simulink model "VTOL_v2"  (R2019b)
settings: Solver=FixedStepAuto  StartTime=0.0  StopTime=inf  FixedStep=Ts  RelTol=1e-3  EnableMultiTasking=on
values from neighbouring files (symbols this model uses):
  k1 = (0.5/axisgains(2) - k2*cruiseThrottle^2)/(cruiseVel^2)    [SensitivityParameterFinder.m]
  k2 = 0.5/(axisgains(2)*hoverpower(1).^2)    [SensitivityParameterFinder.m]
  k3 = (0.5/axisgains(1) - k4*cruiseThrottle^2)/(cruiseVel^2)    [SensitivityParameterFinder.m]
  k4 = 0.5/(axisgains(1)*hoverpower(1).^2)    [SensitivityParameterFinder.m]
  Ts = 1/100    (= 0.01)    [VTOL_params.m]
undefined symbols (not defined in the file or in its folder): color, deltaprops, dev, led_mask, Main, mode, MRC, pwm_output0
libraries: px4uORBlib x13, aerolibutil x8, simulink x6, pwm_sig_converters x4, px4Sensorslib x2, px4lib x2, sharedtransform x2
(part 1 of 3)
settings Model: SimulationMode=external  ExtModeTrigDuration=10  Creator=Robert  LastModifiedBy=Robert
settings SolverCC: PositivePriorityOrder=on  AutoInsertRateTranBlk=on
settings DataIOCC: SaveOutput=off  SignalLogging=off  DSMLogging=off  SaveTime=off  ReturnWorkspaceOutputs=off
settings OptimizationCC: DefaultUnderspecifiedDataType=single  EnhancedBackFolding=on  PassReuseOutputArgsAs=Individual arguments  MaxStackSize=64  OptimizeBlockOrder=speed  DifferentSizesBufferReuse=on  OptimizationCustomize=off  EfficientTunableParamExpr=on
settings DebuggingCC: ParameterTunabilityLossMsg=error  ArithmeticOperatorsInVariantConditions=warning
settings HardwareCC: ProdBitPerPointer=32  ProdBitPerSizeT=32  ProdBitPerPtrDiffT=32  ProdLargestAtomicInteger=Long  ProdLargestAtomicFloat=Double  ProdWordSize=32  ProdLongLongMode=on  ProdHWDeviceType=ARM Compatible->ARM Cortex
settings SFSimCC: MATLABDynamicMemAlloc=off  CustomCodeUndefinedFunction=UseInterfaceOnly
settings RTWCC: SystemTargetFile=ert.tlc  HardwareBoard=PX4 Pixhawk 1  TLCOptions="-aInlineSetEventsForThisBaseRateFcn=TLC_FALSE -aSuppressMultiTaskScheduler=TLC_FALSE  -aRateBasedStepFcn=0"  TemplateMakefile=ert_default_tmf  GenerateReport=on  Toolchain=GNU Tools for PX4 Autopilots  BuildConfiguration=Faster Runs  IncludeHyperlinkInReport=on  LaunchReport=on  TargetLang=C++  GenerateTraceInfo=on  GenerateTraceReport=on  GenerateTraceReportSl=on  GenerateTraceReportSf=on  GenerateTraceReportEml=on
settings CodeAppCC: ForceParamTrailComments=on  IgnoreCustomStorageClasses=off  OperatorAnnotations=on  SimulinkDataObjDesc=on  SFDataObjDesc=on  InsertBlockDesc=on
settings ERTTargetCC: ExtMode=on  ExtModeMexArgs='127.0.0.1' 1 17725

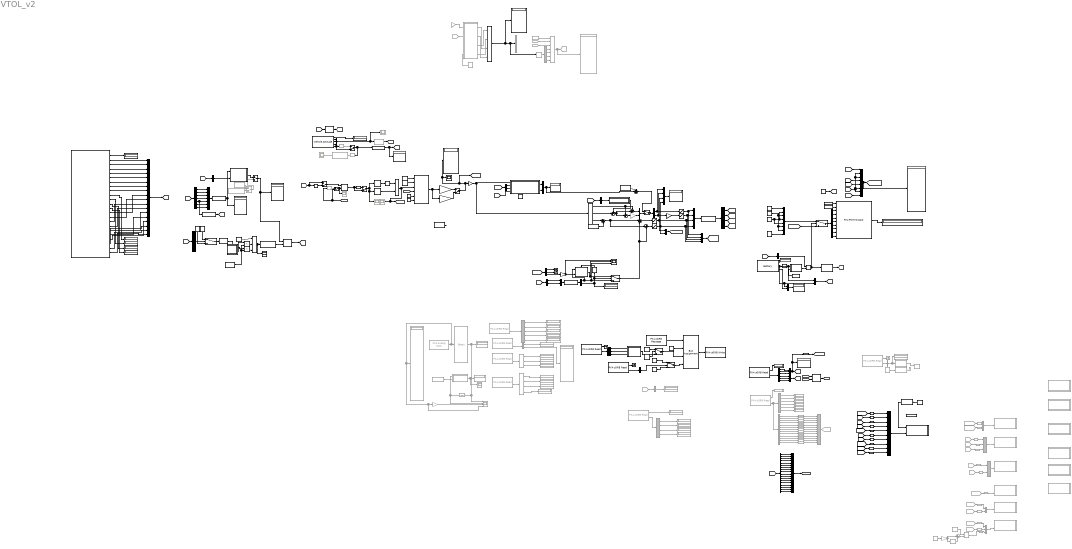
== system VTOL_v2 ==
  note: If SC is touched, initiate step sequence in roll and pitch.
  note: The above needs to match selection in next area;
      | if you run without torque-translator use the top,
      | else the bottom.
  note: Hover requires roughly 0.28 in TL/TR signals.
  note: Old log blocks, MW have given the custgom new ones
  note: The PID parameters for roll/pitch on the single engine one
      | that works are approx
      | [0.6,0,0.015;
      |  0.6,0,0.015]
      |
      | That is, P/D = 40
  note: Some constant pitch torque offset
      | may be necessary due to c.g. z-offset. (No integrators in controller)
  note: Control Area
  note: Before Torque-Translator is used, lets make sure we can hover with this simple linear mixer.
      | Working around the hover point does not need the full range and thus complete non-linear controller.
      | Basic tuning is easier this way - less parameters to adjust.
  note: Part 2 of 2 of the heart of this project.
      | Once the Pixhawk is stable and hover works acceptable this part will be inserted, normalized to not
      | alter the behaviour too much at hover mode, and extend the responses to work well in flying and
      | transition mode as well.
  note: Old translator, only kept for code reference, will never be used.
  note: Crude, ad-hoc, altitude holder for the hover mode.
      | Far from perfect but does the job and frees up one hand to trim/adjust setting etc while hovering.
      | When not holding alt => Pass through
      | throttle stick to joint thrust.
  note: Generate reference quaternion from Transmitter inputs. Very crude reference now, but enough to test stability and do some small steps.
      | Verified in external mode with manual switches.
      |
      | The "mode" (bottom) selects absolute/rate mode
      | on input..
  note: Quaternion extraction from EKF.
      | Handedness verified with manual switches in external mode.
  note: Debug safety switch status
  note: lowpass filter batt voltage for
      | more accurate shutoffs
  note: 3V/cell in LiPo is absolutely the lowest allowed
  note: Make sure model runs at specified frequency
  note: Above (commented out) was a work-around before I got the
      | fixed code for the log block to log at every time step.
  note: Props may not be symmetrical, this offsets the thrust to compensate in that case.
  note: Emergency shutdown switch forces things into
      | off or neutral
  note: Inputs from RC
  note: Outputs, to Servos
  note: Emil Fresk paper on quaternion control, this is part 1 of 2 of the focus on this project. Originally a non-linear attitude controller for
      | multi-rotors, I am trying to use it as a controller for a VTOL fixed wing, non vectored along with a sensitivity normalizer
      | to allow a single controller for hover, transitioning and flying modes.
  note: If either manual emergency stop is pressed or voltage too low cut power.
  note: Logging to SD
  note: Blink LED slowly with Green color on Pixhawk 1
  AND : Logic  Commented=on  IconShape=distinctive  AllPortsSameDT=off  OutDataTypeStr=boolean
  Battery : px4Sensorslib/Battery  voltage=on  current=off  remaining=on  warning=off  timestamp=off  sampleTime=Ts  BlockingMode=off  BlockTimeout=1e-3
      settings: SourceProductName=Embedded Coder Support Package for PX4 Autopilots
  Blink Fast : Constant  Value=5  OutDataTypeStr=Inherit: Inherit via back propagation  SampleTime=1
  Blink Slow : Constant  Value=3  OutDataTypeStr=Inherit: Inherit via back propagation  SampleTime=1
  Bus Assignment : BusAssignment  AssignedSignals=led_mask,color,mode
  Bus Creator : BusCreator  Inputs=18
  Bus Selector : BusSelector  Commented=on  OutputSignals=ch9_SC
  Bus Selector1 : BusSelector  Commented=on  OutputSignals=safety_switch_available,safety_off,override_available,override_enabled
  Bus Selector10 : BusSelector  Commented=on  OutputSignals=fix_type,satellites_used,lat,lon,alt,hdop,vdop,noise_per_ms,jamming_indicator,vel_m_s,vel_n_m_s,vel_e_m_s,vel_d_m_s
  Bus Selector11 : BusSelector  OutputSignals=ch10_SD
  Bus Selector12 : BusSelector  OutputSignals=ch5_S1
  Bus Selector13 : BusSelector  Commented=on  OutputSignals=safety_off
  Bus Selector14 : BusSelector  Commented=on  OutputSignals=channel_value,channel_id
  Bus Selector15 : BusSelector  Commented=on  OutputSignals=hdop,vdop,satellites_used
  Bus Selector16 : BusSelector  Commented=on  OutputSignals=differential_pressure_raw_pa,differential_pressure_filtered_pa,temperature,device_id
  Bus Selector17 : BusSelector  OutputSignals=ch9_SC
  Bus Selector18 : BusSelector  OutputSignals=satellites_used,hdop,vdop
  Bus Selector2 : BusSelector  OutputSignals=ch5_S1
  Bus Selector3 : BusSelector  OutputSignals=ch1_thrust,ch2_Ail,ch3_Ele,ch4_Rud,ch8_SB,ch6_S2,ch7_SA
  Bus Selector4 : BusSelector  OutputSignals=safety_off
  Bus Selector5 : BusSelector  Commented=on  OutputSignals=indicated_airspeed_m_s,true_airspeed_m_s,true_airspeed_unfiltered_m_s,confidence,air_temperature_celsius
  Bus Selector6 : BusSelector  OutputSignals=x,y,z,vx,vy,vz
  Bus Selector7 : BusSelector  OutputSignals=ch1_thrust,ch2_Ail,ch3_Ele,ch4_Rud,ch5_S1,ch6_S2,ch7_SA,ch8_SB,ch9_SC,ch10_SD,ch11_SE,ch12_SF,ch13_SG,ch14_SH,ch15_LS,ch16_RS,ch17_MAX,ch18_MIN
  Bus Selector8 : BusSelector  Commented=on  OutputSignals=lat,lon,alt,satellites_used,hdop,vdop
  Bus Selector9 : BusSelector  OutputSignals=ch1_thrust,ch12_SF
  Cast To Boolean : DataTypeConversion  Commented=on  OutDataTypeStr=boolean
  Cast To Boolean1 : DataTypeConversion  OutDataTypeStr=boolean
  Cast To Boolean2 : DataTypeConversion  OutDataTypeStr=boolean
  Color Amber : Constant  Value=6  OutDataTypeStr=Inherit: Inherit via back propagation  SampleTime=1
  Color Green : Constant  Value=2  OutDataTypeStr=Inherit: Inherit via back propagation  SampleTime=1
  Compare To Zero : simulink/Logic and Bit Operations/Compare To Zero  relop=>  OutDataTypeStr=boolean
  Constant : Constant  Value=logical(1)
  Constant1 : Constant  Value=logical(0)
  Constant10 : Constant  Value=1500  OutDataTypeStr=uint16
  Constant11 : Constant  Value=1500  OutDataTypeStr=uint16
  Constant12 : Constant  Value=1500  OutDataTypeStr=uint16  SampleTime=Ts
  Constant13 : Constant  Commented=on  Value=[cos(pi/4),0,sin(pi/4),0]  SampleTime=Ts
  Constant14 : Constant  Value=boolean(true)  SampleTime=Ts
  Constant15 : Constant  Value=255  OutDataTypeStr=Inherit: Inherit via back propagation  SampleTime=1
  Constant16 : Constant  Commented=on  SampleTime=Ts
  Constant17 : Constant  Value=[3.4,3.4,0.7]'  VectorParams1D=off  SampleTime=Ts
  Constant18 : Constant  Value=0.3  SampleTime=Ts
  Constant19 : Constant  Value=0.6  SampleTime=Ts
  Constant2 : Constant  Commented=on  Value=[0,0,0]  OutDataTypeStr=single  SampleTime=Ts
  Constant20 : Constant  Value=0*0.17.*[1,-1]
  Constant21 : Constant  Commented=on  Value=1.324
  Constant22 : Constant  Value=deg2rad(30)  OutDataTypeStr=single  SampleTime=Ts
  Constant23 : Constant  OutDataTypeStr=single  SampleTime=Ts
  Constant24 : Constant  Value=0  OutDataTypeStr=single  SampleTime=Ts
  Constant25 : Constant  Value=0  OutDataTypeStr=single  SampleTime=Ts
  Constant3 : Constant  Commented=on  Value=0  SampleTime=Ts
  Constant4 : Constant  Value=0.1  SampleTime=Ts
  Constant5 : Constant  Value=0.6  SampleTime=Ts
  Constant6 : Constant  Value=[0,0,0]  SampleTime=Ts
  Constant7 : Constant  Value=1500  OutDataTypeStr=uint16
  Constant8 : Constant  Commented=on  Value=[1,0,0,0]  SampleTime=Ts
  Constant9 : Constant  Value=900  OutDataTypeStr=uint16
  Counter Free-Running : simulink/Sources/Counter Free-Running  Commented=on  NumBits=16  tsamp=Ts
  CutoffVoltage : Constant  Value=3.0*3  OutDataTypeStr=single  SampleTime=Ts
  Data Type Conversion{1..16,20..26,28} (24 alike) : DataTypeConversion  Commented=on  OutDataTypeStr=single
  Data Type Conversion{17,29..30,32..34,36..39,41} (11 alike) : DataTypeConversion  OutDataTypeStr=single
  Data Type Conversion18 : DataTypeConversion  Commented=on  OutDataTypeStr=uint16
  Data Type Conversion19 : DataTypeConversion  Commented=on  OutDataTypeStr=uint16
  Data Type Conversion27 : DataTypeConversion  Commented=on  OutDataTypeStr=double
  Demux : Demux  Outputs=8
  Demux1 : Demux  Commented=on
  Demux2 : Demux  Outputs=2
  Demux4 : Demux  Commented=on
  Demux5 : Demux  Outputs=3
  Demux6 : Demux  Outputs=2
  Demux7 : Demux  Outputs=3
  Demux8 : Demux  Outputs=2
  Demux9 : Demux
  Discrete Transfer Fcn : DiscreteTransferFcn  Numerator=[1-0.99]  Denominator=[1 -0.99]  SampleTime=Ts
  Discrete Transfer Fcn1 : DiscreteTransferFcn  Commented=on  Numerator=[1-0.85]  Denominator=[1 -0.85]  SampleTime=Ts
  Display{,1,3..7,16..21,23..25,28..32,41..51} (32 alike) : Display  Commented=on
  Display{2,8..15,22,26..27,33..40} (20 alike) : Display
      Display9 settings: Format=binary (Stored Integer)
  Divide1 : Product  Commented=on  Inputs=*/
  From11 : From  Commented=on  GotoTag=RC_inputs
  From15 : From  Commented=on  GotoTag=w_bf
  From16 : From  Commented=on  GotoTag=q_bf
  From21 : From  Commented=on  GotoTag=states
  From22 : From  Commented=on  GotoTag=q_ref
  From26 : From  Commented=on  GotoTag=ServoSignals
  From27 : From  Commented=on  GotoTag=mode
  From28 : From  Commented=on  GotoTag=q_wf
  From29 : From  Commented=on  GotoTag=Position
  From30 : From  Commented=on  GotoTag=torques
  From33 : From  Commented=on  GotoTag=axis_err
  From39 : From  Commented=on  GotoTag=volt
  From40 : From  Commented=on  GotoTag=norm_sigs
  From41 : From  Commented=on  GotoTag=stop
  From6 : From  Commented=on  GotoTag=rc_bus
  From7 : From  Commented=on  GotoTag=v_bf
  Gain : Gain  Commented=on  Gain=0.5
  Gain1 : Gain  Commented=on  Gain=18
  Gain2 : Gain
  Gain3 : Gain  Commented=through  Gain=-1
  Gain4 : Gain  Gain=-1
  Gain5 : Gain  Gain=-1
  Gain6 : Gain  Commented=on  Gain=Ts
  Goto11 : Goto  Commented=on  GotoTag=states
  Goto25 : Goto  Commented=on  GotoTag=GPSinfo
  MATLAB Function : MATLAB Function  Commented=on  TreatAsAtomicUnit=on
  MATLAB Function1 : MATLAB Function  TreatAsAtomicUnit=on
  MATLAB Function11 : MATLAB Function  TreatAsAtomicUnit=on
  MATLAB Function12 : MATLAB Function  TreatAsAtomicUnit=on
  MATLAB Function14 : MATLAB Function  TreatAsAtomicUnit=on
  MATLAB Function15 : MATLAB Function  TreatAsAtomicUnit=on
  MATLAB Function16 : MATLAB Function  TreatAsAtomicUnit=on
  MATLAB Function17 : MATLAB Function  Commented=on  TreatAsAtomicUnit=on
  MATLAB Function18 : MATLAB Function  TreatAsAtomicUnit=on
  Manual Switch{,1..3,7} (5 alike) : ManualSwitch  CurrentSetting=0
  Manual Switch4 : ManualSwitch
  Manual Switch5 : ManualSwitch  Commented=on  CurrentSetting=0
  Manual Switch6 : ManualSwitch
  Max : MinMax  Function=max  Inputs=2  OutDataTypeStr=uint16
  Memory : Memory  Commented=on  InheritSampleTime=on
  Memory2 : Memory  Commented=on  InheritSampleTime=on
  Multiply : Product
  Mux : Mux  Inputs=7
  Mux{1,18..20,22,26} (6 alike) : Mux  Inputs=2
  Mux10 : Mux  Commented=on  Inputs=7
  Mux11 : Mux  Commented=on  Inputs=2
  Mux12 : Mux  Commented=on  Inputs=3
  Mux13 : Mux  Commented=on  Inputs=13
  Mux14 : Mux  Inputs=8
  Mux{2,16,24,27} (4 alike) : Mux
  Mux17 : Mux  Commented=on  Inputs=2
  Mux21 : Mux  Inputs=8
  Mux23 : Mux  Commented=on  Inputs=2
  Mux25 : Mux  Commented=on  Inputs=3
  Mux{3,5..7} (4 alike) : Mux  Inputs=3
  Mux4 : Mux  Inputs=10
  Mux8 : Mux  Inputs=18
  PX4 Analog Input : px4lib/PX4 Analog Input  Commented=on  sampleTime=Ts
      settings: SourceProductName=Embedded Coder Support Package for PX4 Autopilots  SourceProductBaseCode=PX4AUTOPILOTS
  PX4 PWM Output : px4lib/PX4 PWM Output  pwmDevice=Main (/dev/pwm_output0)  pwmChannel1_=on  pwmChannel2_=on  pwmChannel3_=on  pwmChannel4_=on  pwmChannel5_=on  pwmChannel6_=on  pwmChannel7_=on  pwmChannel8_=on  forceTerminateFailsafe=off  outputErrorStatus=on
      settings: SourceProductName=Embedded Coder Support Package for PX4 Autopilots
  PX4 SD Card Logger1 : Subsystem  Commented=on  mask(PX4 SD Card Logger){logfile=/fs/microsd/log, logfilename=qlogs, cacheflag=off, numRecs=250*60*60}
      mask prompts: logfile "Log Folder"; logfilename "Log File Name"; cacheflag "Cache in Memory"; numRecs "Maximum Record Count"
      mask help:
      | Log data to a specified file on the SD card
      |
      | The block accepts two inputs, enable and data. The incoming data is logged into the SD card when the enable signal is high and the number of data points logged is less than the Maximum Record Count specified.
      |
      | The specified folder should be present in the SD card for logging.
      |
      | If Cache in Memory is unchecked, the data is written to the SD card at every timestep.  If Cache in Memory is checked, data is cached in the memory and is written to SD card only when enable goes low or when the number of data points logged reaches the Maximum Record Count specified.
      mask init:
      | logname=uint8([logfile,'/',logfilename]);
      mask Help: eval('codertarget.internal.helpView(''px4'',''px4sdcardexample'')');
      mask Display:
      | fprintf([get_param(gcb,'logfile'),'/',get_param(gcb,'logfilename')])
      | port_label('input',1,'en')
      | port_label('input',2,'data')
  PX4 SD Card Logger10 : Subsystem  Commented=on  mask(PX4 SD Card Logger){logfile=/fs/microsd/log, logfilename=MainLog, cacheflag=off, numRecs=MRC}
      mask prompts: logfile "Log Folder"; logfilename "Log File Name"; cacheflag "Cache in Memory"; numRecs "Maximum Record Count"
      mask help:
      | Log data to a specified file on the SD card
      |
      | The block accepts two inputs, enable and data. The incoming data is logged into the SD card when the enable signal is high and the number of data points logged is less than the Maximum Record Count specified.
      |
      | The specified folder should be present in the SD card for logging.
      |
      | If Cache in Memory is unchecked, the data is written to the SD card at every timestep.  If Cache in Memory is checked, data is cached in the memory and is written to SD card only when enable goes low or when the number of data points logged reaches the Maximum Record Count specified.
      mask init:
      | logname=uint8([logfile,'/',logfilename]);
      mask Help: eval('codertarget.internal.helpView(''px4'',''px4sdcardexample'')');
      mask Display:
      | fprintf([get_param(gcb,'logfile'),'/',get_param(gcb,'logfilename')])
      | port_label('input',1,'en')
      | port_label('input',2,'data')
  PX4 SD Card Logger11 : Subsystem  Commented=on  mask(PX4 SD Card Logger){logfile=/fs/microsd/log, logfilename=torques, cacheflag=off, numRecs=MRC}
      mask prompts: logfile "Log Folder"; logfilename "Log File Name"; cacheflag "Cache in Memory"; numRecs "Maximum Record Count"
      mask help:
      | Log data to a specified file on the SD card
      |
      | The block accepts two inputs, enable and data. The incoming data is logged into the SD card when the enable signal is high and the number of data points logged is less than the Maximum Record Count specified.
      |
      | The specified folder should be present in the SD card for logging.
      |
      | If Cache in Memory is unchecked, the data is written to the SD card at every timestep.  If Cache in Memory is checked, data is cached in the memory and is written to SD card only when enable goes low or when the number of data points logged reaches the Maximum Record Count specified.
      mask init:
      | logname=uint8([logfile,'/',logfilename]);
      mask Help: eval('codertarget.internal.helpView(''px4'',''px4sdcardexample'')');
      mask Display:
      | fprintf([get_param(gcb,'logfile'),'/',get_param(gcb,'logfilename')])
      | port_label('input',1,'en')
      | port_label('input',2,'data')
  PX4 SD Card Logger12 : Subsystem  Commented=on  mask(PX4 SD Card Logger){logfile=/fs/microsd/log, logfilename=volt_stop, cacheflag=off, numRecs=MRC}
      mask prompts: logfile "Log Folder"; logfilename "Log File Name"; cacheflag "Cache in Memory"; numRecs "Maximum Record Count"
      mask help:
      | Log data to a specified file on the SD card
      |
      | The block accepts two inputs, enable and data. The incoming data is logged into the SD card when the enable signal is high and the number of data points logged is less than the Maximum Record Count specified.
      |
      | The specified folder should be present in the SD card for logging.
      |
      | If Cache in Memory is unchecked, the data is written to the SD card at every timestep.  If Cache in Memory is checked, data is cached in the memory and is written to SD card only when enable goes low or when the number of data points logged reaches the Maximum Record Count specified.
      mask init:
      | logname=uint8([logfile,'/',logfilename]);
      mask Help: eval('codertarget.internal.helpView(''px4'',''px4sdcardexample'')');
      mask Display:
      | fprintf([get_param(gcb,'logfile'),'/',get_param(gcb,'logfilename')])
      | port_label('input',1,'en')
      | port_label('input',2,'data')
  PX4 SD Card Logger13 : Subsystem  mask(PX4 SD Card Logger){logfile=/fs/microsd/log, logfilename=log, cacheflag=off, numRecs=MRC}
      mask prompts: logfile "Log Folder"; logfilename "Log File Name"; cacheflag "Cache in Memory"; numRecs "Maximum Record Count"
      mask help:
      | Log data to a specified file on the SD card
      |
      | The block accepts two inputs, enable and data. The incoming data is logged into the SD card when the enable signal is high and the number of data points logged is less than the Maximum Record Count specified.
      |
      | The specified folder should be present in the SD card for logging.
      |
      | If Cache in Memory is unchecked, the data is written to the SD card at every timestep.  If Cache in Memory is checked, data is cached in the memory and is written to SD card only when enable goes low or when the number of data points logged reaches the Maximum Record Count specified.
      mask init:
      | logname=uint8([logfile,'/',logfilename]);
      mask Help: eval('codertarget.internal.helpView(''px4'',''px4sdcardexample'')');
      mask Display:
      | fprintf([get_param(gcb,'logfile'),'/',get_param(gcb,'logfilename')])
      | port_label('input',1,'en')
      | port_label('input',2,'data')
  PX4 SD Card Logger2 : Subsystem  Commented=on  mask(PX4 SD Card Logger){logfile=/fs/microsd/log, logfilename=rc_and_servosignals, cacheflag=off, numRecs=250*60*60}
      mask prompts: logfile "Log Folder"; logfilename "Log File Name"; cacheflag "Cache in Memory"; numRecs "Maximum Record Count"
      mask help:
      | Log data to a specified file on the SD card
      |
      | The block accepts two inputs, enable and data. The incoming data is logged into the SD card when the enable signal is high and the number of data points logged is less than the Maximum Record Count specified.
      |
      | The specified folder should be present in the SD card for logging.
      |
      | If Cache in Memory is unchecked, the data is written to the SD card at every timestep.  If Cache in Memory is checked, data is cached in the memory and is written to SD card only when enable goes low or when the number of data points logged reaches the Maximum Record Count specified.
      mask init:
      | logname=uint8([logfile,'/',logfilename]);
      mask Help: eval('codertarget.internal.helpView(''px4'',''px4sdcardexample'')');
      mask Display:
      | fprintf([get_param(gcb,'logfile'),'/',get_param(gcb,'logfilename')])
      | port_label('input',1,'en')
      | port_label('input',2,'data')
  PX4 SD Card Logger3 : Subsystem  Commented=on  mask(PX4 SD Card Logger){logfile=/fs/microsd/log, logfilename=norm_sigs, cacheflag=off, numRecs=250*60*60}
      mask prompts: logfile "Log Folder"; logfilename "Log File Name"; cacheflag "Cache in Memory"; numRecs "Maximum Record Count"
      mask help:
      | Log data to a specified file on the SD card
      |
      | The block accepts two inputs, enable and data. The incoming data is logged into the SD card when the enable signal is high and the number of data points logged is less than the Maximum Record Count specified.
      |
      | The specified folder should be present in the SD card for logging.
      |
      | If Cache in Memory is unchecked, the data is written to the SD card at every timestep.  If Cache in Memory is checked, data is cached in the memory and is written to SD card only when enable goes low or when the number of data points logged reaches the Maximum Record Count specified.
      mask init:
      | logname=uint8([logfile,'/',logfilename]);
      mask Help: eval('codertarget.internal.helpView(''px4'',''px4sdcardexample'')');
      mask Display:
      | fprintf([get_param(gcb,'logfile'),'/',get_param(gcb,'logfilename')])
      | port_label('input',1,'en')
      | port_label('input',2,'data')
  PX4 SD Card Logger4 : Subsystem  Commented=on  mask(PX4 SD Card Logger){logfile=/fs/microsd/log, logfilename=MainLog, cacheflag=off, numRecs=250*60*60}
      mask prompts: logfile "Log Folder"; logfilename "Log File Name"; cacheflag "Cache in Memory"; numRecs "Maximum Record Count"
      mask help:
      | Log data to a specified file on the SD card
      |
      | The block accepts two inputs, enable and data. The incoming data is logged into the SD card when the enable signal is high and the number of data points logged is less than the Maximum Record Count specified.
      |
      | The specified folder should be present in the SD card for logging.
      |
      | If Cache in Memory is unchecked, the data is written to the SD card at every timestep.  If Cache in Memory is checked, data is cached in the memory and is written to SD card only when enable goes low or when the number of data points logged reaches the Maximum Record Count specified.
      mask init:
      | logname=uint8([logfile,'/',logfilename]);
      mask Help: eval('codertarget.internal.helpView(''px4'',''px4sdcardexample'')');
      mask Display:
      | fprintf([get_param(gcb,'logfile'),'/',get_param(gcb,'logfilename')])
      | port_label('input',1,'en')
      | port_label('input',2,'data')
  PX4 SD Card Logger5 : Subsystem  Commented=on  mask(PX4 SD Card Logger){logfile=/fs/microsd/log, logfilename=torques, cacheflag=off, numRecs=250*60*60}
      mask prompts: logfile "Log Folder"; logfilename "Log File Name"; cacheflag "Cache in Memory"; numRecs "Maximum Record Count"
      mask help:
      | Log data to a specified file on the SD card
      |
      | The block accepts two inputs, enable and data. The incoming data is logged into the SD card when the enable signal is high and the number of data points logged is less than the Maximum Record Count specified.
      |
      | The specified folder should be present in the SD card for logging.
      |
      | If Cache in Memory is unchecked, the data is written to the SD card at every timestep.  If Cache in Memory is checked, data is cached in the memory and is written to SD card only when enable goes low or when the number of data points logged reaches the Maximum Record Count specified.
      mask init:
      | logname=uint8([logfile,'/',logfilename]);
      mask Help: eval('codertarget.internal.helpView(''px4'',''px4sdcardexample'')');
      mask Display:
      | fprintf([get_param(gcb,'logfile'),'/',get_param(gcb,'logfilename')])
      | port_label('input',1,'en')
      | port_label('input',2,'data')
  PX4 SD Card Logger6 : Subsystem  Commented=on  mask(PX4 SD Card Logger){logfile=/fs/microsd/log, logfilename=volt_stop, cacheflag=off, numRecs=250*60*60}
      mask prompts: logfile "Log Folder"; logfilename "Log File Name"; cacheflag "Cache in Memory"; numRecs "Maximum Record Count"
      mask help:
      | Log data to a specified file on the SD card
      |
      | The block accepts two inputs, enable and data. The incoming data is logged into the SD card when the enable signal is high and the number of data points logged is less than the Maximum Record Count specified.
      |
      | The specified folder should be present in the SD card for logging.
      |
      | If Cache in Memory is unchecked, the data is written to the SD card at every timestep.  If Cache in Memory is checked, data is cached in the memory and is written to SD card only when enable goes low or when the number of data points logged reaches the Maximum Record Count specified.
      mask init:
      | logname=uint8([logfile,'/',logfilename]);
      mask Help: eval('codertarget.internal.helpView(''px4'',''px4sdcardexample'')');
      mask Display:
      | fprintf([get_param(gcb,'logfile'),'/',get_param(gcb,'logfilename')])
      | port_label('input',1,'en')
      | port_label('input',2,'data')
  PX4 SD Card Logger7 : Subsystem  Commented=on  mask(PX4 SD Card Logger){logfile=/fs/microsd/log, logfilename=qlogs, cacheflag=off, numRecs=MRC}
      mask prompts: logfile "Log Folder"; logfilename "Log File Name"; cacheflag "Cache in Memory"; numRecs "Maximum Record Count"
      mask help:
      | Log data to a specified file on the SD card
      |
      | The block accepts two inputs, enable and data. The incoming data is logged into the SD card when the enable signal is high and the number of data points logged is less than the Maximum Record Count specified.
      |
      | The specified folder should be present in the SD card for logging.
      |
      | If Cache in Memory is unchecked, the data is written to the SD card at every timestep.  If Cache in Memory is checked, data is cached in the memory and is written to SD card only when enable goes low or when the number of data points logged reaches the Maximum Record Count specified.
      mask init:
      | logname=uint8([logfile,'/',logfilename]);
      mask Help: eval('codertarget.internal.helpView(''px4'',''px4sdcardexample'')');
      mask Display:
      | fprintf([get_param(gcb,'logfile'),'/',get_param(gcb,'logfilename')])
      | port_label('input',1,'en')
      | port_label('input',2,'data')
  PX4 SD Card Logger8 : Subsystem  Commented=on  mask(PX4 SD Card Logger){logfile=/fs/microsd/log, logfilename=rc_and_servosignals, cacheflag=off, numRecs=MRC}
      mask prompts: logfile "Log Folder"; logfilename "Log File Name"; cacheflag "Cache in Memory"; numRecs "Maximum Record Count"
      mask help:
      | Log data to a specified file on the SD card
      |
      | The block accepts two inputs, enable and data. The incoming data is logged into the SD card when the enable signal is high and the number of data points logged is less than the Maximum Record Count specified.
      |
      | The specified folder should be present in the SD card for logging.
      |
      | If Cache in Memory is unchecked, the data is written to the SD card at every timestep.  If Cache in Memory is checked, data is cached in the memory and is written to SD card only when enable goes low or when the number of data points logged reaches the Maximum Record Count specified.
      mask init:
      | logname=uint8([logfile,'/',logfilename]);
      mask Help: eval('codertarget.internal.helpView(''px4'',''px4sdcardexample'')');
      mask Display:
      | fprintf([get_param(gcb,'logfile'),'/',get_param(gcb,'logfilename')])
      | port_label('input',1,'en')
      | port_label('input',2,'data')
  PX4 SD Card Logger9 : Subsystem  Commented=on  mask(PX4 SD Card Logger){logfile=/fs/microsd/log, logfilename=norm_sigs, cacheflag=off, numRecs=MRC}
      mask prompts: logfile "Log Folder"; logfilename "Log File Name"; cacheflag "Cache in Memory"; numRecs "Maximum Record Count"
      mask help:
      | Log data to a specified file on the SD card
      |
      | The block accepts two inputs, enable and data. The incoming data is logged into the SD card when the enable signal is high and the number of data points logged is less than the Maximum Record Count specified.
      |
      | The specified folder should be present in the SD card for logging.
      |
      | If Cache in Memory is unchecked, the data is written to the SD card at every timestep.  If Cache in Memory is checked, data is cached in the memory and is written to SD card only when enable goes low or when the number of data points logged reaches the Maximum Record Count specified.
      mask init:
      | logname=uint8([logfile,'/',logfilename]);
      mask Help: eval('codertarget.internal.helpView(''px4'',''px4sdcardexample'')');
      mask Display:
      | fprintf([get_param(gcb,'logfile'),'/',get_param(gcb,'logfilename')])
      | port_label('input',1,'en')
      | port_label('input',2,'data')
  PX4 uORB Message : px4uORBlib/PX4 uORB Message  uORBTopic=led_control  SampleTime=inf
      settings: SourceProductName=Embedded Coder Support Package for PX4 Autopilots  SourceProductBaseCode=PX4AUTOPILOTS
  PX4 uORB Read : px4uORBlib/PX4 uORB Read  uORBTopic=vehicle_local_position  sampleTime=Ts  BlockingMode=off  BlockTimeout=1e-3
      settings: SourceProductName=Embedded Coder Support Package for PX4 Autopilots
  PX4 uORB Read1 : px4uORBlib/PX4 uORB Read  Commented=on  uORBTopic=safety  sampleTime=Ts  BlockingMode=off  BlockTimeout=1e-3
      settings: SourceProductName=Embedded Coder Support Package for PX4 Autopilots
  PX4 uORB Read2 : px4uORBlib/PX4 uORB Read  Commented=on  uORBTopic=vehicle_gps_position  sampleTime=0.004  BlockingMode=off  BlockTimeout=1e-3
      settings: SourceProductName=Embedded Coder Support Package for PX4 Autopilots
  PX4 uORB Read3 : px4uORBlib/PX4 uORB Read  Commented=on  uORBTopic=safety  sampleTime=Ts  BlockingMode=off  BlockTimeout=1e-3
      settings: SourceProductName=Embedded Coder Support Package for PX4 Autopilots
  PX4 uORB Read4 : px4uORBlib/PX4 uORB Read  uORBTopic=safety  sampleTime=1  BlockingMode=off  BlockTimeout=1e-3
      settings: SourceProductName=Embedded Coder Support Package for PX4 Autopilots
  PX4 uORB Read5 : px4uORBlib/PX4 uORB Read  Commented=on  uORBTopic=airspeed  sampleTime=Ts  BlockingMode=off  BlockTimeout=1e-3
      settings: SourceProductName=Embedded Coder Support Package for PX4 Autopilots  SourceProductBaseCode=PX4AUTOPILOTS
  PX4 uORB Read6 : px4uORBlib/PX4 uORB Read  Commented=on  uORBTopic=adc_report  sampleTime=Ts  BlockingMode=off  BlockTimeout=1e-3
      settings: SourceProductName=Embedded Coder Support Package for PX4 Autopilots  SourceProductBaseCode=PX4AUTOPILOTS
  PX4 uORB Read7 : px4uORBlib/PX4 uORB Read  Commented=on  uORBTopic=vehicle_gps_position  sampleTime=Ts  BlockingMode=off  BlockTimeout=1e-3
      settings: SourceProductName=Embedded Coder Support Package for PX4 Autopilots  SourceProductBaseCode=PX4AUTOPILOTS
  PX4 uORB Read8 : px4uORBlib/PX4 uORB Read  Commented=on  uORBTopic=differential_pressure  sampleTime=Ts  BlockingMode=off  BlockTimeout=1e-3
      settings: SourceProductName=Embedded Coder Support Package for PX4 Autopilots  SourceProductBaseCode=PX4AUTOPILOTS
  PX4 uORB Read9 : px4uORBlib/PX4 uORB Read  uORBTopic=vehicle_gps_position  sampleTime=1  BlockingMode=off  BlockTimeout=1e-3
      settings: SourceProductName=Embedded Coder Support Package for PX4 Autopilots  SourceProductBaseCode=PX4AUTOPILOTS
  PX4 uORB Write : px4uORBlib/PX4 uORB Write  uORBTopic=led_control  MessageQueueLen=1
      settings: SourceProductName=Embedded Coder Support Package for PX4 Autopilots  SourceProductBaseCode=PX4AUTOPILOTS
  Product : Product
  Product1 : Product
  PropOffset : Constant  Value=deltaprops  OutDataTypeStr=single  SampleTime=Ts
  Pulse Generator : DiscretePulseGenerator  Commented=on  SampleTime=Ts
  Pulse Generator1 : DiscretePulseGenerator  Period=3  SampleTime=Ts
  Quaternion Conjugate1 : aerolibutil/Quaternion Conjugate
      settings: SourceProductName=Aerospace Blockset  SourceProductBaseCode=AE
  Quaternion Conjugate10 : aerolibutil/Quaternion Conjugate
      settings: SourceProductName=Aerospace Blockset  SourceProductBaseCode=AE
  Quaternion Conjugate2 : aerolibutil/Quaternion Conjugate  Commented=on
      settings: SourceProductName=Aerospace Blockset  SourceProductBaseCode=AE
  Quaternion Conjugate7 : aerolibutil/Quaternion Conjugate  Commented=on
      settings: SourceProductName=Aerospace Blockset  SourceProductBaseCode=AE
  Quaternion Conjugate8 : aerolibutil/Quaternion Conjugate
      settings: SourceProductName=Aerospace Blockset  SourceProductBaseCode=AE
  Quaternion Multiplication : aerolibutil/Quaternion Multiplication
  Quaternion Multiplication1 : aerolibutil/Quaternion Multiplication
  Quaternion Rotation4 : aerolibutil/Quaternion Rotation
  Quaternions to Rotation Angles1 : sharedtransform/Quaternions to Rotation Angles  Commented=on  rotationOrder=ZYX  aMode=aMode
      settings: SourceProductBaseCode=AE
  Radio Control Transmitter : Subsystem  AncestorBlock=px4Sensorslib/Radio Control Transmitter  mask(PX4 Radio Control Transmitter){channel1=on, channel2=on, channel3=on, channel4=on, channel5=on, channel6=on, channel7=on, channel8=on, channel_count=on, rssi=on, rc_input_source=on, timestamp_last_signal=on, time_stamp=off, sampleTime=Ts, BlockingMode=off, BlockTimeout=5}
      mask prompts: channel1 "px4:blockmask:uORBRCBlockMaskCh1"; channel2 "px4:blockmask:uORBRCBlockMaskCh2"; channel3 "px4:blockmask:uORBRCBlockMaskCh3"; channel4 "px4:blockmask:uORBRCBlockMaskCh4"; channel5 "px4:blockmask:uORBRCBlockMaskCh5"; channel6 "px4:blockmask:uORBRCBlockMaskCh6"; channel7 "px4:blockmask:uORBRCBlockMaskCh7"; channel8 "px4:blockmask:uORBRCBlockMaskCh8"; channel_count "px4:blockmask:uORBRCBlockMaskChCount"; rssi "px4:blockmask:uORBRCBlockMaskRSSI"; rc_input_source "px4:blockmask:uORBRCBlockMaskRCSource"; timestamp_last_signal "px4:blockmask:uORBRCBlockMaskRCTimestampLastSignal"; time_stamp "px4:blockmask:uORBRCBlockMaskTs"; sampleTime "px4:blockmask:SampleTimePrompt"; BlockingMode "px4:blockmask:SubscriberBlockingMode"; BlockTimeout "px4:blockmask:SubscriberBlockingModeTimeout"
      mask help: px4:blockmask:uORBRCBlockMaskDescription
      mask init:
      | signal_names = {'channel_1','channel_2','channel_3','channel_4',...
      |                         'channel_5','channel_6','channel_7','channel_8',...
      |                         '<channel_count>','<rssi>',...
      |                         '<input_source>','<timestamp_last_signal>','<timestamp>'};
      | output_port_names = {'Ch 1','Ch 2','Ch 3',...
      |                         'Ch 4','Ch 5','Ch 6','Ch 7',...
      |                         'Ch 8','Num Ch','RSSI',...
      |                         'RC Source','Last valid time','Timestamp'...
      |                         };
      | mask_image = 'mask_input_rc.png';                    
      | imfilename = fullfile(codertarget.pixhawk.internal.getSpPkgRootDir, 'resources', mask_image);
      | px4.internal.block.CommonuORBTopicMask.commonMaskCallback(gcb,signal_names,output_port_names,imfilename);
      mask Help: eval('codertarget.internal.helpView(''px4'',''px4librctransmitter'')');
      mask TypeOptions sampleTime: PX4 uORB Read/sampleTime
      mask TypeOptions BlockingMode: PX4 uORB Read/BlockingMode
      mask Callback BlockingMode: px4.internal.block.CommonuORBTopicMask.blockingModeCallback(gcb);
      mask TypeOptions BlockTimeout: PX4 uORB Read/BlockTimeout
      mask DialogControl Container10 Prompt: px4:blockmask:uORBRCBlockMainTab
      mask DialogControl Container14 Prompt: px4:blockmask:uORBRCBlockChSelection
      mask DialogControl channel1 Prompt: Channel 1
      mask DialogControl channel2 Prompt: Channel 2
      mask DialogControl channel3 Prompt: Channel 3
      mask DialogControl channel4 Prompt: Channel 4
      mask DialogControl channel5 Prompt: Channel 5
      mask DialogControl channel6 Prompt: Channel 6
      mask DialogControl channel7 Prompt: Channel 7
      mask DialogControl channel8 Prompt: Channel 8
      mask DialogControl Container17 Prompt: px4:blockmask:uORBRCBlockAdditionalOp
      mask DialogControl channel_count Prompt: Number of channels actually being seen
      mask DialogControl rssi Prompt: Receive signal strength indicator (RSSI)
      mask DialogControl rc_input_source Prompt: Radio control input source
      mask DialogControl timestamp_last_signal Prompt: Last valid reception time (in us)
      mask DialogControl time_stamp Prompt: Timestamp (in us)
      mask DialogControl sampleTime Prompt: Sample time (-1 for inherited):
      mask DialogControl Container19 Prompt: px4:blockmask:uORBRCBlockAdvancedTab
      mask DialogControl BlockingMode Prompt: Wait until data received
      mask DialogControl BlockTimeout Prompt: Timeout in seconds:
      mask Display:
      | color('white');
      | plot([100,100,100,100],[100,100,100,100]);
      | plot([0,0,0,0],[0,0,0,0]);
      | image('C:\ProgramData\MATLAB\SupportPackages\R2019b\toolbox\target\supportpackages\px4\resources\mask_input_rc.png','center')
      | color('blue');
      | text(0.25, 0.9, 'PX4', 'horizontalAlignment', 'right');
      | color('black');
      | port_label('output',1,'Status');
      | port_label('output',2,'Ch 1');
      | port_label('output',3,'Ch 2');
      | port_label('output',4,'Ch 3');
      | port_label('output',5,'Ch 4');
      | port_label('output',6,'Ch 5');
      | port_label('output',7,'Ch 6');
      | port_label('output',8,'Ch 7');
      | port_label('output',9,'Ch 8');
      | port_label('output',10,'Num Ch');
      | port_label('output',11,'RSSI');
      | port_label('output',12,'RC Source');
      | port_label('output',13,'Last valid time');
  Rotation Angles to Quaternions : sharedtransform/Rotation Angles to Quaternions  rotationOrder=ZYX  aMode=aMode
      settings: SourceProductName=Aerospace Blockset  SourceProductBaseCode=AE
  Saturation{,1..3} (4 alike) : Saturate  UpperLimit=1  LowerLimit=-1
  Scope : Scope  NumInputPorts=3
  Scope{1,4..6,25,35} (6 alike) : Scope  Commented=on
  Scope2 : Scope  Commented=on  NumInputPorts=4
  Scope3 : Scope
  Scope7 : Scope
  Selector : Selector  Commented=on  InputPortWidth=12  IndexOptions=Index vector (dialog)  Indices=[9]  OutputSizes=1
  Selector2 : Selector  IndexMode=Zero-based  InputPortWidth=4  IndexOptions=Index vector (dialog)  Indices=[0 ]  OutputSizes=1
  Selector3 : Selector  IndexMode=Zero-based  InputPortWidth=4  IndexOptions=Index vector (dialog)  Indices=[1:3]  OutputSizes=1
  Sign : Signum
  Signal Specification1 : SignalSpecification  OutDataTypeStr=single
  Subsystem : Subsystem
  Subsystem1 : Subsystem
  Sum : Sum  Inputs=++|
  Sum2 : Sum  Inputs=-+|
  Sum3 : Sum  Inputs=++|
  Sum4 : Sum  Inputs=|++
  Sum5 : Sum  Inputs=|-+
  Sum6 : Sum  Inputs=++|
  Sum7 : Sum  Inputs=|++
  Sum9 : Sum  Commented=on  Inputs=|+-
  Switch : Switch  Criteria=u2 > Threshold
  Switch1 : Switch  Criteria=u2 > Threshold  Threshold=1300
  Switch2 : Switch  Criteria=u2 > Threshold  Threshold=0.5
  Switch3 : Switch  Criteria=u2 > Threshold  Threshold=1300
  Switch4 : Switch  Criteria=u2 > Threshold
  Terminator{,1,3..4} (4 alike) : Terminator
  Terminator2 : Terminator  Commented=on
  TorqueTranslator : MATLAB Function  Commented=on  TreatAsAtomicUnit=on
  Transfer Fcn First Order1 : simulink/Discrete/Transfer Fcn First Order  Commented=through  PoleZ=0.9  ICPrevOutput=0.0  DoSatur=off
      settings: SourceProductName=Simulink
  Vehicle Attitude1 : px4Sensorslib/Vehicle Attitude  rollRate=on  pitchRate=on  yawRate=on  quaternion=on  uorbTimeStamp=off  BlockingMode=off  BlockTimeout=0.001  sampleTime=Ts
      settings: SourceProductName=Embedded Coder Support Package for PX4 Autopilots
  "axisgains " : Gain  Gain=[3.4,3.4,0.7]
  pwm2sig : pwm_sig_converters/pwm2sig  SystemSampleTime=-1  Latency=0  AutoFrameSizeCalculation=off
  pwm2sig1 : pwm_sig_converters/pwm2sig  SystemSampleTime=-1  Latency=0  AutoFrameSizeCalculation=off
  pwm2sig2 : pwm_sig_converters/pwm2sig  SystemSampleTime=-1  Latency=0  AutoFrameSizeCalculation=off
  sig2pwm : pwm_sig_converters/sig2pwm  SystemSampleTime=-1  Latency=0  AutoFrameSizeCalculation=off
  torqueTranslatorGains : Gain  Gain=[1,1,0.7]
  wires:
  Demux1/4 -> Mux10/7
  Quaternion Conjugate7/1 -> Manual Switch/1
  Demux6/2 -> Display37/1, Switch/2, Compare To Zero/1
  Bus Selector7/10 -> Mux8/10  "<ch10_SD>"
  Sum3/1 -> Gain3/1
  Demux7/2 -> Terminator1/1
  Multiply/1 -> [axis_err], Scope4/1, MATLAB Function11/3(angErr)
  Battery/3 -> Mux22/2
  Demux5/1 -> Sum2/1, Sum3/1  "tao_x"
  [rc_bus] -> Bus Selector11/1
  Switch1/1 -> Demux/1
  Compare To Zero/1 -> Subsystem/Enable
  Battery/2 -> Discrete Transfer Fcn/1, Mux26/2, Mux22/1
  Demux/8 -> PX4 PWM Output/10
  Data Type Conversion8/1 -> Mux13/5
  Constant11/1 -> Mux21/8
  Mux2/1 -> Memory/1, Demux4/1, Display10/1
  Bus Selector/1 -> Display/1  "<ch9_SC>"
  Demux9/2 -> [ElevonR]
  Demux1/2 -> Mux10/5
  Constant7/1 -> Mux21/1
  Demux/1 -> PX4 PWM Output/3
  Constant9/1 -> Mux21/2, Mux21/4, Mux21/5
  Bus Selector7/2 -> Mux8/2  "<ch2_Ail>"
  Quaternion Multiplication/1 -> Quaternion Conjugate10/1, Manual Switch3/2  "qerr_wf"
  Demux7/3 -> Gain4/1
  Demux9/4 -> [ThrustR]
  [ServoSignals] -> Switch1/3
  Bus Selector10/2 -> Data Type Conversion5/1  "<satellites_used>"
  Mux20/1 -> Sum/2, Display38/1
  Max/1 -> MATLAB Function18/1(u), Switch1/2
  Sum6/1 -> Sum3/2, Sum2/2
  Bus Selector7/3 -> Mux8/3  "<ch3_Ele>"
  Bus Selector10/6 -> Data Type Conversion9/1  "<hdop>"
  Data Type Conversion6/1 -> Mux13/3
  Subsystem/1("throttle ") -> Switch/1, Scope/2
  Constant10/1 -> Mux21/7, Mux21/6, Mux21/3
  Bus Selector6/5 -> Mux7/2  "<vy>"
  MATLAB Function15/1(stopsig) -> Max/2
  Demux8/1 -> MATLAB Function14/2(u_omegaL)
  Bus Selector3/5 -> pwm2sig2/1, Mux/5  "<ch8_SB>"
  Data Type Conversion9/1 -> Mux13/6
  Bus Selector8/4 -> Display21/1  "<satellites_used>"
  TorqueTranslator/3(u_deltaL) -> Mux2/1  "uWL"
  Bus Selector10/10 -> Data Type Conversion13/1  "<vel_m_s>"
  Manual Switch1/1 -> Quaternion Multiplication/1
  Bus Selector6/1 -> Mux5/1  "<x>"
  PX4 PWM Output/1 -> Display9/1
  Demux2/2 -> Mux16/2, Gain5/1
  Gain2/1 -> MATLAB Function14/1(tao), Demux5/1
  Bus Selector3/6 -> Mux/6  "<ch6_S2>"
  Bus Selector9/1 -> Mux18/1  "<ch1_thrust>"
  Switch/1 -> Sum4/2, Sum5/2
  Mux22/1 -> Display39/1
  Bus Selector11/1 -> Max/1  "<ch10_SD>"
  Demux6/1 -> Subsystem/1(throttle), Switch/3, Scope/3
  Bus Selector1/3 -> Display6/1  "<override_available>"
  Demux/4 -> PX4 PWM Output/6
  Demux8/2 -> MATLAB Function14/3(u_omegaR)
  Data Type Conversion7/1 -> Mux13/4
  [u_omegas] -> Demux8/1
  Bus Selector10/9 -> Data Type Conversion12/1  "<jamming_indicator>"
  [q_wf] -> Manual Switch/2, Quaternion Conjugate7/1  "qerr_bf"
  Sum7/1 -> Sum5/1, Sum4/1
  Demux/3 -> PX4 PWM Output/5
  Manual Switch4/1 -> Quaternion Multiplication1/1, Display36/1
  [Position] -> Demux7/1
  Constant2/1 -> Mux10/1
  Bus Selector8/1 -> Display29/1  "<lat>"
  Mux21/1 -> Switch1/1
  Manual Switch3/1 -> Scope35/1, Selector3/1, Selector2/1
  Mux19/1 -> [u_omegas]
  [w_bf] -> MATLAB Function11/4(w)
  Bus Selector7/8 -> Mux8/8  "<ch8_SB>"
  Sign/1 -> Multiply/1  "rotdir"
  Data Type Conversion16/1 -> Mux13/13
  Gain4/1 -> Scope/1, Subsystem/2(alt)
  Vehicle Attitude1/5 -> Manual Switch2/2, Quaternion Conjugate2/1
  Vehicle Attitude1/4 -> Mux6/3
  [ElevonR] -> Mux14/1
  TorqueTranslator/4(u_deltaR) -> Mux2/2  "udeltaL"
  Vehicle Attitude1/2 -> Mux6/1
  Bus Selector1/1 -> Display4/1  "<safety_switch_available>"
  Quaternion Conjugate1/1 -> [q_bf]
  Constant17/1 -> ?
  PX4 uORB Read1/2 -> Bus Selector1/1
  pwm2sig1/1 -> MATLAB Function12/1(sticks), Display35/1
  [rc_bus] -> Bus Selector3/1
  Demux9/3 -> [ThrustL]
  Bus Selector10/11 -> Data Type Conversion14/1  "<vel_n_m_s>"
  Bus Selector6/4 -> Mux7/1  "<vx>"
  Bus Selector3/3 -> Mux/3  "<ch3_Ele>"
  Bus Selector3/1 -> Mux/1  "<ch1_thrust>"
  Bus Selector10/8 -> Data Type Conversion11/1  "<noise_per_ms>"
  Demux9/1 -> [ElevonL]
  Data Type Conversion14/1 -> Mux13/11
  Bus Selector10/12 -> Data Type Conversion15/1  "<vel_e_m_s>"
  Bus Selector7/15 -> Mux8/15  "<ch15_LS>"
  Data Type Conversion12/1 -> Mux13/9
  Data Type Conversion13/1 -> Mux13/10
  Bus Selector7/9 -> Mux8/9  "<ch9_SC>"
  [ThrustL] -> Mux14/5
  Data Type Conversion10/1 -> Mux13/7
  Data Type Conversion5/1 -> Mux13/2
  Demux/6 -> PX4 PWM Output/8
  Selector3/1 -> Multiply/2  "axiserr"
  Demux/7 -> PX4 PWM Output/9
  Mux7/1 -> [v_wf]
  Mux14/1 -> Display8/1, [ServoSignals]
  [Others] -> Mux14/2, Mux14/3, Mux14/6, Mux14/7
  Bus Selector7/12 -> Mux8/12  "<ch12_SF>"
  Bus Selector7/14 -> Mux8/14  "<ch14_SH>"
  Bus Selector7/11 -> Mux8/11  "<ch11_SE>"
  Bus Selector10/1 -> Data Type Conversion4/1  "<fix_type>"
  [rc_bus] -> Bus Selector7/1
  Bus Selector7/6 -> Mux8/6  "<ch6_S2>"
  Bus Selector10/13 -> Data Type Conversion16/1  "<vel_d_m_s>"
  TorqueTranslator/2(u_omegaR) -> Mux2/4
  Bus Selector7/7 -> Mux8/7  "<ch7_SA>"
  [q_wf] -> Quaternion Conjugate1/1
  Manual Switch/1 -> Scope25/1, Quaternion Multiplication/2
  Bus Selector7/18 -> Mux8/18  "<ch18_MIN>"
  Mux16/1 -> Display33/1
  Selector2/1 -> Sign/1  "q0"
  Demux2/1 -> Mux16/1, Saturation/1
  From16/1 -> Mux10/3  "q"
  [q_ref] -> Manual Switch1/1, Quaternion Conjugate8/1
  Vehicle Attitude1/3 -> Mux6/2
  Constant4/1 -> MATLAB Function11/2(D)
  Gain1/1 -> TorqueTranslator/1(u_jointT)
  Data Type Conversion17/1 -> [Position]
  Constant5/1 -> MATLAB Function11/1(P)
  Manual Switch7/1 -> Display27/1, Scope7/1, [torques], Gain2/1
  PX4 uORB Read1/1 -> Display1/1
  [v_wf] -> Quaternion Rotation4/2
  Bus Selector7/4 -> Mux8/4  "<ch4_Rud>"
  Bus Selector7/17 -> Mux8/17  "<ch17_MAX>"
  Bus Selector1/2 -> Display5/1  "<safety_off>"
  Sum5/1 -> Saturation3/1
  Bus Selector9/2 -> Mux18/2  "<ch12_SF>"
  Constant3/1 -> TorqueTranslator/4(pitchoffset)
  From21/1 -> TorqueTranslator/2(states)
  Demux/2 -> PX4 PWM Output/4
  Bus Selector7/16 -> Mux8/16  "<ch16_RS>"
  Memory/1 -> Demux1/1
  Data Type Conversion11/1 -> Mux13/8
  Sum4/1 -> Saturation2/1
  From15/1 -> Mux10/2  "w"
  TorqueTranslator/1(u_omegaL) -> Mux2/3  "uWL"
  [ElevonL] -> Mux14/8
  MATLAB Function14/2(u_deltaR) -> Mux20/2
  pwm2sig2/1 -> [mode]
  PX4 uORB Read/1 -> Display34/1
  [ThrustR] -> Mux14/4
  Bus Selector10/4 -> Data Type Conversion7/1  "<lon>"
  Bus Selector3/2 -> Mux/2  "<ch2_Ail>"
  Data Type Conversion4/1 -> Mux13/1
  Quaternion Rotation4/1 -> [v_bf]
  Signal Specification1/1 -> Display22/1, [q_wf]
  Vehicle Attitude1/1 -> Display26/1
  Bus Selector6/3 -> Mux5/3  "<z>"
  Bus Selector8/2 -> Display30/1  "<lon>"
  PX4 uORB Read/2 -> Bus Selector6/1
  CutoffVoltage/1 -> MATLAB Function15/2(cutoff)
  Bus Selector7/1 -> Mux8/1  "<ch1_thrust>"
  Battery/1 -> Display40/1
  [q_bf] -> Quaternion Rotation4/1
  Mux8/1 -> [RC_inputs]
  Bus Selector10/3 -> Data Type Conversion6/1  "<lat>"
  PX4 uORB Read2/1 -> Display32/1
  Mux18/1 -> pwm2sig/1
  MATLAB Function14/1(u_deltaL) -> Mux20/1
  Demux7/1 -> Terminator/1
  Constant1/1 -> PX4 PWM Output/2
  Bus Creator/1 -> [rc_bus]
  Bus Selector1/4 -> Display7/1  "<override_enabled>"
  Bus Selector6/6 -> Mux7/3  "<vz>"
  Constant/1 -> PX4 PWM Output/1
  Constant12/1 -> [Others]
  Bus Selector7/5 -> Mux8/5  "<ch5_S1>"
  Demux1/1 -> Mux10/4
  Radio Control Transmitter/1(Out_Status) -> Display14/1
  From6/1 -> Bus Selector/1
  PX4 uORB Read2/2 -> Bus Selector10/1, Bus Selector8/1
  Mux/1 -> pwm2sig1/1
  Quaternion Conjugate8/1 -> Manual Switch1/2
  Bus Selector10/5 -> Data Type Conversion8/1  "<alt>"
  Demux1/3 -> Mux10/6
  Bus Selector6/2 -> Mux5/2  "<y>"
  Mux13/1 -> Goto25/1
  Bus Selector7/13 -> Mux8/13  "<ch13_SG>"
  Mux5/1 -> Data Type Conversion17/1, Display2/1, [r_wf]
  pwm2sig/1 -> Demux6/1
  Mux10/1 -> Display31/1, Goto11/1
  Bus Selector10/7 -> Data Type Conversion10/1  "<vdop>"
  Data Type Conversion15/1 -> Mux13/12
  [rc_bus] -> Bus Selector9/1
  Bus Selector3/4 -> Mux/4  "<ch4_Rud>"
  Bus Selector8/5 -> Display23/1  "<hdop>"
  Demux/5 -> PX4 PWM Output/7
  Bus Selector8/3 -> Display28/1  "<alt>"
  Bus Selector8/6 -> Display20/1  "<vdop>"
  Saturation/1 -> Mux27/1, Mux24/1
  Saturation1/1 -> Mux27/2, Mux24/2
  Saturation2/1 -> Mux19/1, Mux16/3, Mux27/3, Mux24/3
  Saturation3/1 -> Mux19/2, Mux16/4, Mux27/4, Mux24/4
  Demux5/2 -> Sum6/2  "tao_y"
  MATLAB Function16/1(offset) -> Sum6/1
  Bus Selector3/7 -> Mux/7  "<ch7_SA>"
  [rc_bus] -> Bus Selector2/1
  Bus Selector2/1 -> MATLAB Function12/2(offset_stick)  "<ch5_S1>"
  Transfer Fcn First Order1/1 -> [w_bf]
  Bus Selector12/1 -> MATLAB Function16/1(offset_stick)  "<ch5_S1>"
  [rc_bus] -> Bus Selector12/1
  PX4 uORB Read3/2 -> Bus Selector13/1
  Bus Selector13/1 -> MATLAB Function17/1(u), Display41/1  "<safety_off>"
  Mux24/1 -> [norm_sigs]
  Demux5/3 -> Sum7/1  "tao_z"
  PropOffset/1 -> Sum7/2
  MATLAB Function17/1(y) -> AND/1
  From22/1 -> Data Type Conversion21/1
  Data Type Conversion23/1 -> Mux23/1
  From30/1 -> Data Type Conversion23/1
  From27/1 -> Data Type Conversion2/1
  From11/1 -> Data Type Conversion18/1
  Data Type Conversion2/1 -> Mux12/1
  From26/1 -> Data Type Conversion19/1
  Data Type Conversion18/1 -> Mux11/1
  From33/1 -> Data Type Conversion25/1
  From28/1 -> Data Type Conversion3/1
  Data Type Conversion19/1 -> Mux11/2
  From29/1 -> Data Type Conversion20/1
  From40/1 -> Data Type Conversion24/1
  Data Type Conversion20/1 -> Mux12/2
  Mux17/1 -> PX4 SD Card Logger7/2(Data)
  Mux11/1 -> PX4 SD Card Logger8/2(Data)
  Mux23/1 -> PX4 SD Card Logger11/2(Data)
  Data Type Conversion24/1 -> PX4 SD Card Logger9/2(Data)
  Data Type Conversion21/1 -> Mux17/2
  Mux12/1 -> PX4 SD Card Logger10/2(Data)
  Data Type Conversion3/1 -> Mux17/1
  Data Type Conversion25/1 -> Mux23/2
  Pulse Generator/1 -> Cast To Boolean/1
  Cast To Boolean/1 -> ?
  Mux25/1 -> PX4 SD Card Logger12/2(Data)
  Data Type Conversion26/1 -> Mux25/2
  ? -> PX4 SD Card Logger8/1(En), PX4 SD Card Logger10/1(En), PX4 SD Card Logger7/1(En), PX4 SD Card Logger9/1(En), PX4 SD Card Logger12/1(En), PX4 SD Card Logger11/1(En)
  From41/1 -> Data Type Conversion26/1
  Data Type Conversion22/1 -> Mux25/1
  From39/1 -> Data Type Conversion22/1
  MATLAB Function18/1(y) -> [stop]
  PX4 uORB Read3/1 -> Terminator2/1
  Discrete Transfer Fcn/1 -> MATLAB Function15/1(voltage), Mux26/1
  Mux26/1 -> [volt]
  Quaternion Conjugate2/1 -> Manual Switch2/1
  Manual Switch2/1 -> Data Type Conversion27/1, Signal Specification1/1
  Mux6/1 -> Scope5/1, Transfer Fcn First Order1/1
  Quaternions to Rotation Angles1/1 -> Scope6/1
  Data Type Conversion27/1 -> Quaternions to Rotation Angles1/1
  Quaternion Conjugate10/1 -> Manual Switch3/1
  Manual Switch5/1 -> Manual Switch4/2
  MATLAB Function12/1(q_ref) -> Manual Switch4/1
  Constant13/1 -> Manual Switch5/2
  Constant8/1 -> Manual Switch5/1
  Divide1/1 -> Data Type Conversion28/1
  Sum9/1 -> Divide1/2
  Constant16/1 -> Divide1/1
  Memory2/1 -> Sum9/2
  Gain6/1 -> Sum9/1, Memory2/1
  Data Type Conversion28/1 -> Mux25/3
  sig2pwm/1 -> Demux9/1
  Mux27/1 -> sig2pwm/1
  Radio Control Transmitter/2(Outport_channel1) -> Bus Creator/1  "ch1_thrust"
  Radio Control Transmitter/3(Outport_channel2) -> Bus Creator/2  "ch2_Ail"
  Radio Control Transmitter/4(Outport_channel3) -> Bus Creator/3  "ch3_Ele"
  Radio Control Transmitter/5(Outport_channel4) -> Bus Creator/4  "ch4_Rud"
  Radio Control Transmitter/6(Outport_channel5) -> Bus Creator/5  "ch5_S1"
  Radio Control Transmitter/7(Outport_channel6) -> Bus Creator/6  "ch6_S2"
  Radio Control Transmitter/8(Outport_channel7) -> Bus Creator/7  "ch7_SA"
  Radio Control Transmitter/9(Outport_channel8) -> Bus Creator/8  "ch8_SB"
  Radio Control Transmitter/18(Outport_channel13) -> Bus Creator/13  "ch13_SG"
  Radio Control Transmitter/19(Outport_channel14) -> Bus Creator/14  "ch14_SH"
  Radio Control Transmitter/14(Outport_channel9) -> Bus Creator/9  "ch9_SC"
  Radio Control Transmitter/15(Outport_channel10) -> Bus Creator/10  "ch10_SD"
  Radio Control Transmitter/13(Outport_timestamp_last_signal) -> Display13/1  "Last Valid TIme"
  Radio Control Transmitter/12(Outport_rc_input_source) -> Display15/1  "RC Source"
  Radio Control Transmitter/11(Outport_rssi) -> Display12/1  "RSSI"
  Radio Control Transmitter/10(Outport_channel_count) -> Display11/1  "num ch"
  Radio Control Transmitter/16(Outport_channel11) -> Bus Creator/11  "ch11_SE"
  Radio Control Transmitter/17(Outport_channel12) -> Bus Creator/12  "ch12_SF"
  Radio Control Transmitter/20(Outport_channel15) -> Bus Creator/15  "ch15_LS"
  Radio Control Transmitter/21(Outport_channel16) -> Bus Creator/16  "ch16_RS"
  Radio Control Transmitter/22(Outport_channel17) -> Bus Creator/17  "ch17_MAX"
  Radio Control Transmitter/23(Outport_channel18) -> Bus Creator/18  "ch18_MIN"
  PX4 uORB Message/1 -> Bus Assignment/1
  Constant15/1 -> Bus Assignment/2
  Bus Assignment/1 -> PX4 uORB Write/1
  Blink Fast/1 -> Switch2/1
  Blink Slow/1 -> Switch2/3
  PX4 uORB Read4/1 -> Terminator3/1
  Switch2/1 -> Bus Assignment/4
  PX4 uORB Read4/2 -> Bus Selector4/1
  Bus Selector4/1 -> Switch2/2  "<safety_off>"
  Constant19/1 -> MATLAB Function11/5(PZ)
  Constant18/1 -> MATLAB Function11/6(DZ)
  Sum2/1 -> Mux1/1
  Gain3/1 -> Mux1/2
  Mux1/1 -> Manual Switch6/2
  Manual Switch6/1 -> Demux2/1
  "axisgains "/1 -> Manual Switch7/1
  torqueTranslatorGains/1 -> Manual Switch7/2
  MATLAB Function11/1(taos) -> torqueTranslatorGains/1, "axisgains "/1
  Sum/1 -> Manual Switch6/1
  Constant20/1 -> Sum/1
  Gain5/1 -> Saturation1/1
  From7/1 -> Data Type Conversion1/1
  Data Type Conversion1/1 -> Mux12/3
  [v_bf] -> MATLAB Function14/4(v)
  PX4 uORB Read5/2 -> Bus Selector5/1
  PX4 uORB Read6/2 -> Bus Selector14/1
  PX4 uORB Read7/2 -> Bus Selector15/1
  Bus Selector15/1 -> Display3/1  "<hdop>"
  Bus Selector15/2 -> Display16/1  "<vdop>"
  Bus Selector15/3 -> Display17/1  "<satellites_used>"
  Bus Selector14/1 -> Display18/1  "<channel_value>"
  Bus Selector14/2 -> Display19/1  "<channel_id>"
  Bus Selector5/1 -> Display24/1  "<indicated_airspeed_m_s>"
  Bus Selector5/2 -> Display25/1  "<true_airspeed_m_s>"
  Bus Selector5/3 -> Display42/1  "<true_airspeed_unfiltered_m_s>"
  Bus Selector5/4 -> Display43/1  "<confidence>"
  Bus Selector5/5 -> Display44/1  "<air_temperature_celsius>"
  PX4 uORB Read8/2 -> Bus Selector16/1
  Bus Selector16/1 -> Display47/1  "<differential_pressure_raw_pa>"
  Bus Selector16/2 -> Display45/1  "<differential_pressure_filtered_pa>"
  Bus Selector16/3 -> Display46/1  "<temperature>"
  Bus Selector16/4 -> Display48/1  "<device_id>"
  Selector/1 -> Display49/1, Scope2/1, Discrete Transfer Fcn1/1
  MATLAB Function/1(airspeed) -> Scope1/1, Display50/1
  Constant21/1 -> MATLAB Function/2(zeroSignal)
  Discrete Transfer Fcn1/1 -> Scope2/2, MATLAB Function/1(ADC)
  PX4 Analog Input/1 -> Scope2/4, Gain/1, Display51/1, Selector/1
  Gain/1 -> Scope2/3
  [rc_bus] -> Bus Selector17/1
  Bus Selector17/1 -> Switch3/2  "<ch9_SC>"
  Switch3/1 -> Cast To Boolean1/1
  Constant23/1 -> Switch3/1
  Constant24/1 -> Switch3/3
  Constant25/1 -> Mux3/1
  Subsystem1/2(pitchstep) -> Product1/1
  Subsystem1/1(rollstep) -> Product/1
  Mux3/1 -> Scope3/1, Rotation Angles to Quaternions/1
  Rotation Angles to Quaternions/1 -> Quaternion Multiplication1/2
  Quaternion Multiplication1/1 -> [q_ref]
  Cast To Boolean1/1 -> Subsystem1/Enable
  Product/1 -> Mux3/3
  Product1/1 -> Mux3/2
  Constant22/1 -> Product1/2, Product/2
  PX4 uORB Read9/2 -> Bus Selector18/1
  PX4 uORB Read9/1 -> Terminator4/1
  Color Green/1 -> Switch4/1
  Color Amber/1 -> Switch4/3
  Switch4/1 -> Bus Assignment/3
  Bus Selector18/1 -> MATLAB Function1/1(sats)  "<satellites_used>"
  Bus Selector18/2 -> MATLAB Function1/2(hdop)  "<hdop>"
  Bus Selector18/3 -> MATLAB Function1/3(vdop)  "<vdop>"
  MATLAB Function1/1(gps_good) -> Switch4/2
  Counter Free-Running/1 -> Gain6/1
  Data Type Conversion34/1 -> Mux4/7
  [axis_err] -> Data Type Conversion38/1
  [RC_inputs] -> Data Type Conversion30/1
  [stop] -> Data Type Conversion39/1
  [norm_sigs] -> Data Type Conversion37/1
  [mode] -> Data Type Conversion32/1
  [v_bf] -> Data Type Conversion29/1
  [q_wf] -> Data Type Conversion41/1
  Data Type Conversion41/1 -> Mux4/6
  [Position] -> Data Type Conversion33/1
  Data Type Conversion37/1 -> Mux4/5
  [q_ref] -> Data Type Conversion34/1
  Data Type Conversion30/1 -> Mux4/1
  [torques] -> Data Type Conversion36/1
  Data Type Conversion32/1 -> Mux4/2
  Data Type Conversion33/1 -> Mux4/3
  Data Type Conversion29/1 -> Mux4/4
  Data Type Conversion36/1 -> Mux4/8
  Data Type Conversion38/1 -> Mux4/9
  Data Type Conversion39/1 -> Mux4/10
  Mux4/1 -> PX4 SD Card Logger13/2(Data)
  Cast To Boolean2/1 -> PX4 SD Card Logger13/1(En)
  Pulse Generator1/1 -> Cast To Boolean2/1
